simulink model "estimator_de_stare"  (R2023b)
settings: Solver=VariableStepAuto  StartTime=0.0  StopTime=1000  RelTol=1e-3
settings Model: Creator=Iustin  LastModifiedBy=Iustin

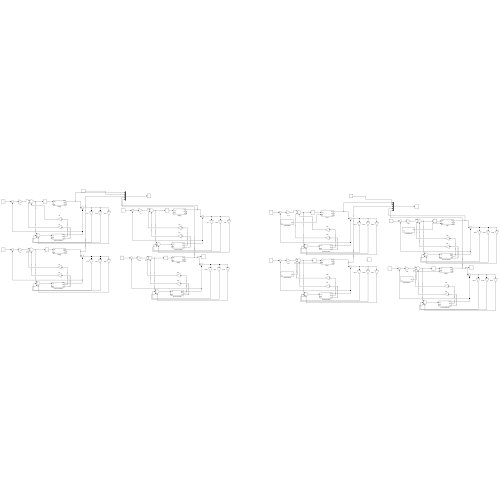
[thumbnail: Simulink's stored preview of the top-level diagram]
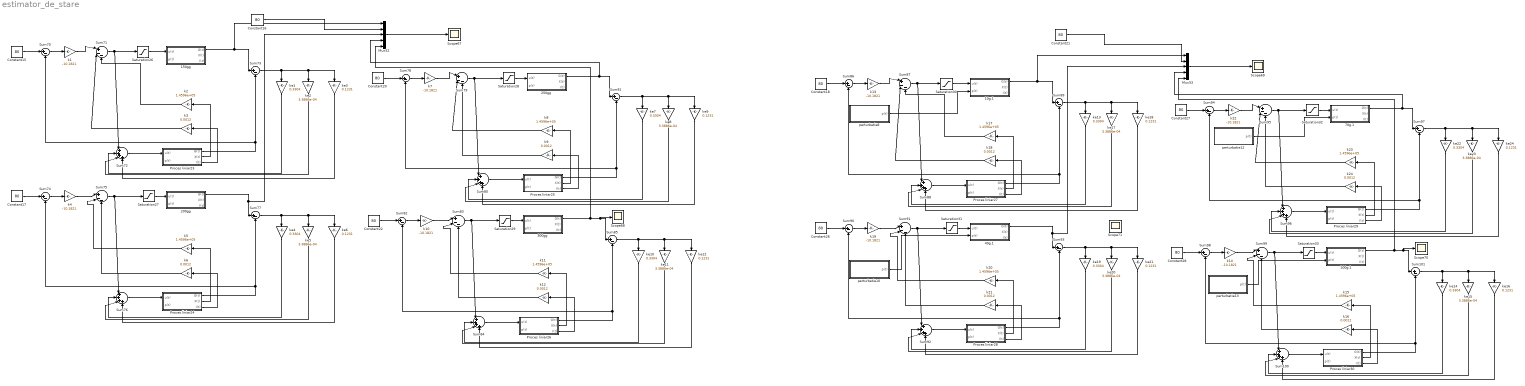
== system estimator_de_stare ==
  " Proces liniar23" : Subsystem  mask{p1=0.005, p2=0.017, p3=0.00000808, n=0.175, V=120, Gb=80, G0=100, Xb=0.0054}
  " Proces liniar24" : Subsystem  mask{p1=0.005, p2=0.017, p3=0.00000808, n=0.175, V=120, Gb=80, G0=100, Xb=0.0054}
  " Proces liniar25" : Subsystem  mask{p1=0.005, p2=0.017, p3=0.00000808, n=0.175, V=120, Gb=80, G0=100, Xb=0.0054}
  " Proces liniar26" : Subsystem  mask{p1=0.005, p2=0.017, p3=0.00000808, n=0.175, V=120, Gb=80, G0=100, Xb=0.0054}
  " Proces liniar27" : Subsystem  mask{p1=0.005, p2=0.017, p3=0.00000808, n=0.175, V=120, Gb=80, G0=100, Xb=0.0054}
  " Proces liniar28" : Subsystem  mask{p1=0.005, p2=0.017, p3=0.00000808, n=0.175, V=120, Gb=80, G0=100, Xb=0.0054}
  " Proces liniar29" : Subsystem  mask{p1=0.005, p2=0.017, p3=0.00000808, n=0.175, V=120, Gb=80, G0=100, Xb=0.0054}
  " Proces liniar30" : Subsystem  mask{p1=0.005, p2=0.017, p3=0.00000808, n=0.175, V=120, Gb=80, G0=100, Xb=0.0054}
  100g.1 : Subsystem  mask{p1=0.005, p2=0.017, p3=0.00000808, n=0.175, V=120, Gb=80, G0=100}
  10g.1 : Subsystem  mask{p1=0.005, p2=0.017, p3=0.00000808, n=0.175, V=120, Gb=80, G0=100}
  150gg : Subsystem  mask{p1=0.005, p2=0.017, p3=0.00000808, n=0.175, V=120, Gb=80, G0=150}
  200gg : Subsystem  mask{p1=0.005, p2=0.017, p3=0.00000808, n=0.175, V=120, Gb=80, G0=200}
  250gg : Subsystem  mask{p1=0.005, p2=0.017, p3=0.00000808, n=0.175, V=120, Gb=80, G0=250}
  300gg : Subsystem  mask{p1=0.005, p2=0.017, p3=0.00000808, n=0.175, V=120, Gb=80, G0=300}
  40g.1 : Subsystem  mask{p1=0.005, p2=0.017, p3=0.00000808, n=0.175, V=120, Gb=80, G0=100}
  70g.1 : Subsystem  mask{p1=0.005, p2=0.017, p3=0.00000808, n=0.175, V=120, Gb=80, G0=100}
  Constant{15..18,20..22,26..28} (10 alike) : Constant  Value=80
  Mux52 : Mux  Inputs=5
  Mux53 : Mux  Inputs=5
  Saturation{26..33} (8 alike) : Saturate  UpperLimit=500  LowerLimit=0
  Scope{67..71} (5 alike) : Scope
  Sum{72,76,80,84,88,92,96,100} (8 alike) : Sum  Inputs=|++++
  Sum{70,73..74,77..78,81..82,85..86,89..90,93..94,97..98,101} (16 alike) : Sum  Inputs=|+-
  Sum{71,75,79,83,87,91,95,99} (8 alike) : Sum  Inputs=|+--
  k{1,4,7,10,13..14,19,22} (8 alike) : Gain  Gain=-10.1821
  k{2,5,8,11,15,17,20,23} (8 alike) : Gain  Gain=1.4596e+05
  k{3,6,9,12,16,18,21,24} (8 alike) : Gain  Gain=0.0012
  ke{1,4,7,10,13..14,19,22} (8 alike) : Gain  Gain=0.3304
  ke{2,5,8,11,15,17,20,23} (8 alike) : Gain  Gain=3.3886e-04
  ke{3,6,9,12,16,18,21,24} (8 alike) : Gain  Gain=0.1231
  perturbatie10 : Subsystem  mask{Dg=40*1000, Ag=0.8, tg_max=40}
  perturbatie12 : Subsystem  mask{Dg=70*1000, Ag=0.8, tg_max=40}
  perturbatie13 : Subsystem  mask{Dg=100*1000, Ag=0.8, tg_max=40}
  perturbatie8 : Subsystem  mask{Dg=10*1000, Ag=0.8, tg_max=40}
  wires:
  ke17/1 -> Sum88/3
  ke19/1 -> Sum92/2
  k23/1 -> Sum95/2
  ke15/1 -> Sum100/3
  " Proces liniar28"/2(X(t)) -> k20/1
  " Proces liniar27"/1(" G(t)") -> Sum86/2, Sum89/2
  k17/1 -> Sum87/3
  " Proces liniar25"/2(X(t)) -> k8/1
  Constant18/1 -> Sum86/1
  " Proces liniar25"/3(I(t)) -> k9/1
  perturbatie10/1(p(t)) -> 40g.1/2(p(t))
  " Proces liniar26"/1(" G(t)") -> Sum82/2, Sum85/2
  k15/1 -> Sum99/2
  k22/1 -> Sum95/1
  ke2/1 -> Sum72/3
  k8/1 -> Sum79/2
  ke13/1 -> Sum88/2
  ke5/1 -> Sum76/3
  40g.1/1(" G(t)") -> Mux53/3, Sum93/1
  Sum75/1 -> Saturation27/1, Sum76/1
  Constant20/1 -> Sum78/1
  k11/1 -> Sum83/2
  Constant15/1 -> Sum70/1
  Constant28/1 -> Sum98/1
  " Proces liniar28"/3(I(t)) -> k21/1
  " Proces liniar29"/1(" G(t)") -> Sum94/2, Sum97/2
  ke7/1 -> Sum80/2
  10g.1/1(" G(t)") -> Mux53/1, Sum89/1
  Sum74/1 -> k4/1
  Sum86/1 -> k13/1
  Sum95/1 -> Saturation32/1, Sum96/1
  perturbatie13/1(p(t)) -> 100g.1/2(p(t))
  perturbatie12/1(p(t)) -> 70g.1/2(p(t))
  Sum93/1 -> ke19/1, ke20/1, ke21/1
  perturbatie8/1(p(t)) -> 10g.1/2(p(t))
  " Proces liniar27"/2(X(t)) -> k17/1
  Sum82/1 -> k10/1
  k19/1 -> Sum91/1
  ke14/1 -> Sum100/2
  " Proces liniar25"/1(" G(t)") -> Sum78/2, Sum81/2
  Constant26/1 -> Sum90/1
  Saturation31/1 -> 40g.1/1(" u(t)")
  ke22/1 -> Sum96/2
  ke20/1 -> Sum92/3
  ke10/1 -> Sum84/2
  k3/1 -> Sum71/2
  Constant27/1 -> Sum94/1
  Saturation32/1 -> 70g.1/1(" u(t)")
  ke23/1 -> Sum96/3
  Sum92/1 -> " Proces liniar28"/1(" u(t)")
  Sum88/1 -> " Proces liniar27"/1(" u(t)")
  " Proces liniar29"/3(I(t)) -> k24/1
  " Proces liniar27"/3(I(t)) -> k18/1
  Constant16/1 -> Mux52/2
  Saturation33/1 -> 100g.1/1(" u(t)")
  k21/1 -> Sum91/3
  k16/1 -> Sum99/3
  " Proces liniar29"/2(X(t)) -> k23/1
  Sum91/1 -> Saturation31/1, Sum92/1
  k9/1 -> Sum79/3
  Sum100/1 -> " Proces liniar30"/1(" u(t)")
  Sum89/1 -> ke13/1, ke17/1, ke18/1
  k6/1 -> Sum75/3
  ke24/1 -> Sum96/4
  ke21/1 -> Sum92/4
  ke16/1 -> Sum100/4
  Sum94/1 -> k22/1
  " Proces liniar30"/3(I(t)) -> k16/1
  Sum99/1 -> Saturation33/1, Sum100/1
  " Proces liniar30"/1(" G(t)") -> Sum98/2, Sum101/2
  k20/1 -> Sum91/2
  k24/1 -> Sum95/3
  Sum101/1 -> ke14/1, ke15/1, ke16/1
  Sum87/1 -> Saturation30/1, Sum88/1
  ke11/1 -> Sum84/3
  Mux53/1 -> Scope69/1
  k18/1 -> Sum87/2
  300gg/1(" G(t)") -> Mux52/5, Scope68/1, Sum85/1
  150gg/1(" G(t)") -> Mux52/1, Sum73/1
  k14/1 -> Sum99/1
  100g.1/1(" G(t)") -> Mux53/5, Scope70/1, Sum101/1
  k12/1 -> Sum83/3
  Sum77/1 -> ke4/1, ke5/1, ke6/1
  ke4/1 -> Sum76/2
  ke6/1 -> Sum76/4
  " Proces liniar24"/2(X(t)) -> k5/1
  Sum97/1 -> ke22/1, ke23/1, ke24/1
  Saturation27/1 -> 200gg/1(" u(t)")
  Constant17/1 -> Sum74/1
  ke12/1 -> Sum84/4
  " Proces liniar24"/3(I(t)) -> k6/1
  Sum98/1 -> k14/1
  Constant21/1 -> Mux53/2
  " Proces liniar26"/2(X(t)) -> k11/1
  " Proces liniar23"/1(" G(t)") -> Sum70/2, Sum73/2
  ke18/1 -> Sum88/4
  " Proces liniar28"/1(" G(t)") -> Sum90/2, Sum93/2
  " Proces liniar23"/2(X(t)) -> k2/1
  Sum76/1 -> " Proces liniar24"/1(" u(t)")
  Saturation30/1 -> 10g.1/1(" u(t)")
  200gg/1(" G(t)") -> Mux52/3, Sum77/1
  Sum90/1 -> k19/1
  " Proces liniar23"/3(I(t)) -> k3/1
  Sum71/1 -> Saturation26/1, Sum72/1
  Mux52/1 -> Scope67/1
  k5/1 -> Sum75/2
  k1/1 -> Sum71/1
  Sum70/1 -> k1/1
  Saturation28/1 -> 250gg/1(" u(t)")
  " Proces liniar26"/3(I(t)) -> k12/1
  Saturation29/1 -> 300gg/1(" u(t)")
  Sum84/1 -> " Proces liniar26"/1(" u(t)")
  70g.1/1(" G(t)") -> Mux53/4, Sum97/1
  Sum85/1 -> ke10/1, ke11/1, ke12/1
  " Proces liniar30"/2(X(t)) -> k15/1
  Sum73/1 -> ke1/1, ke2/1, ke3/1
  k2/1 -> Sum71/3
  Sum96/1 -> " Proces liniar29"/1(" u(t)")
  ke9/1 -> Sum80/4
  Constant22/1 -> Sum82/1
  k10/1 -> Sum83/1
  Sum78/1 -> k7/1
  ke3/1 -> Sum72/4
  Sum80/1 -> " Proces liniar25"/1(" u(t)")
  Saturation26/1 -> 150gg/1(" u(t)")
  ke8/1 -> Sum80/3
  Sum81/1 -> ke7/1, ke8/1, ke9/1
  Sum79/1 -> Saturation28/1, Sum80/1
  k13/1 -> Sum87/1
  Sum83/1 -> Saturation29/1, Sum84/1
  250gg/1(" G(t)") -> Mux52/4, Sum81/1
  ke1/1 -> Sum72/2
  " Proces liniar24"/1(" G(t)") -> Sum74/2, Sum77/2
  k4/1 -> Sum75/1
  k7/1 -> Sum79/1
  Sum72/1 -> " Proces liniar23"/1(" u(t)")

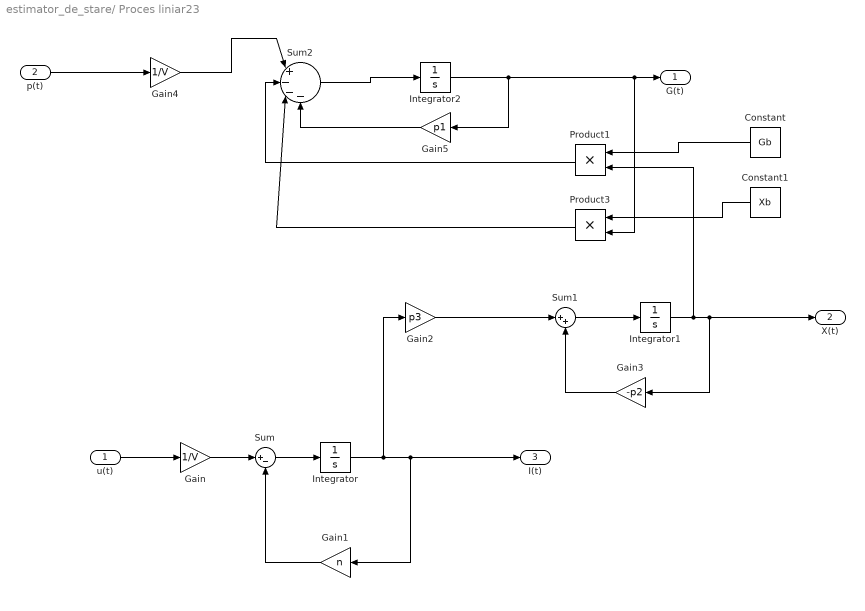
== system estimator_de_stare/ Proces liniar23 ==
  " u(t)" : Inport
  p(t) : Inport  Port=2
  Constant : Constant  Value=Gb
  Constant1 : Constant  Value=Xb
  Gain : Gain  Gain=1/V
  Gain1 : Gain  Gain=n
  Gain2 : Gain  Gain=p3
  Gain3 : Gain  Gain=-p2
  Gain4 : Gain  Gain=1/V
  Gain5 : Gain  Gain=p1
  Integrator : Integrator
  Integrator1 : Integrator
  Integrator2 : Integrator  InitialCondition=G0
  Product1 : Product
  Product3 : Product
  Sum : Sum  Inputs=|+-
  Sum1 : Sum  Inputs=|++
  Sum2 : Sum  Inputs=|+---
  " G(t)" : Outport
  X(t) : Outport  Port=2
  I(t) : Outport  Port=3
  wires:
  Gain2/1 -> Sum1/1
  Gain/1 -> Sum/1
  " u(t)"/1 -> Gain/1
  Sum/1 -> Integrator/1
  Gain1/1 -> Sum/2
  Integrator2/1 -> Product3/2, " G(t)"/1, Gain5/1
  Integrator1/1 -> Product1/2, Gain3/1, X(t)/1
  Integrator/1 -> Gain2/1, I(t)/1, Gain1/1
  Gain3/1 -> Sum1/2
  Gain4/1 -> Sum2/1
  Gain5/1 -> Sum2/4
  p(t)/1 -> Gain4/1
  Sum1/1 -> Integrator1/1
  Sum2/1 -> Integrator2/1
  Constant/1 -> Product1/1
  Constant1/1 -> Product3/1
  Product3/1 -> Sum2/3
  Product1/1 -> Sum2/2

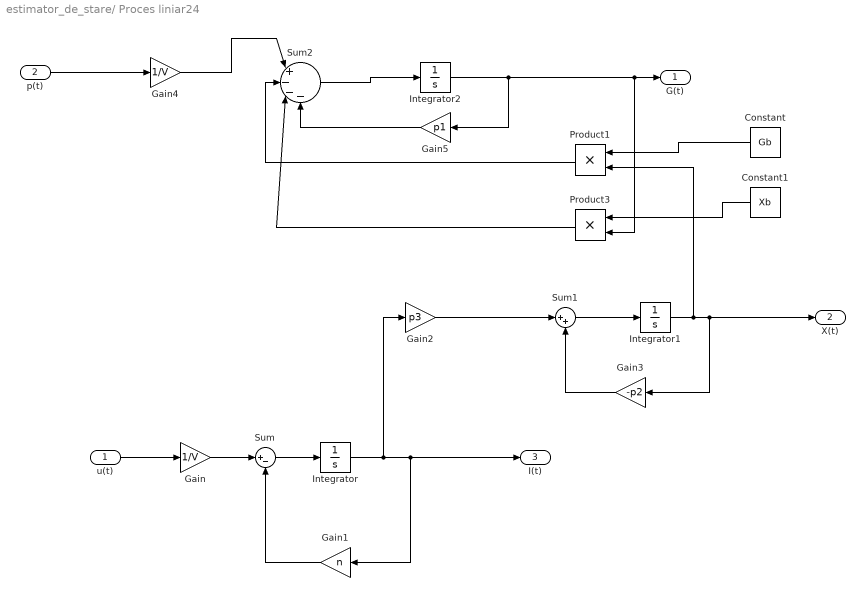
== system estimator_de_stare/ Proces liniar24 ==
  " u(t)" : Inport
  p(t) : Inport  Port=2
  Constant : Constant  Value=Gb
  Constant1 : Constant  Value=Xb
  Gain : Gain  Gain=1/V
  Gain1 : Gain  Gain=n
  Gain2 : Gain  Gain=p3
  Gain3 : Gain  Gain=-p2
  Gain4 : Gain  Gain=1/V
  Gain5 : Gain  Gain=p1
  Integrator : Integrator
  Integrator1 : Integrator
  Integrator2 : Integrator  InitialCondition=G0
  Product1 : Product
  Product3 : Product
  Sum : Sum  Inputs=|+-
  Sum1 : Sum  Inputs=|++
  Sum2 : Sum  Inputs=|+---
  " G(t)" : Outport
  X(t) : Outport  Port=2
  I(t) : Outport  Port=3
  wires:
  Gain2/1 -> Sum1/1
  Gain/1 -> Sum/1
  " u(t)"/1 -> Gain/1
  Sum/1 -> Integrator/1
  Gain1/1 -> Sum/2
  Integrator2/1 -> Product3/2, " G(t)"/1, Gain5/1
  Integrator1/1 -> Product1/2, Gain3/1, X(t)/1
  Integrator/1 -> Gain2/1, I(t)/1, Gain1/1
  Gain3/1 -> Sum1/2
  Gain4/1 -> Sum2/1
  Gain5/1 -> Sum2/4
  p(t)/1 -> Gain4/1
  Sum1/1 -> Integrator1/1
  Sum2/1 -> Integrator2/1
  Constant/1 -> Product1/1
  Constant1/1 -> Product3/1
  Product3/1 -> Sum2/3
  Product1/1 -> Sum2/2

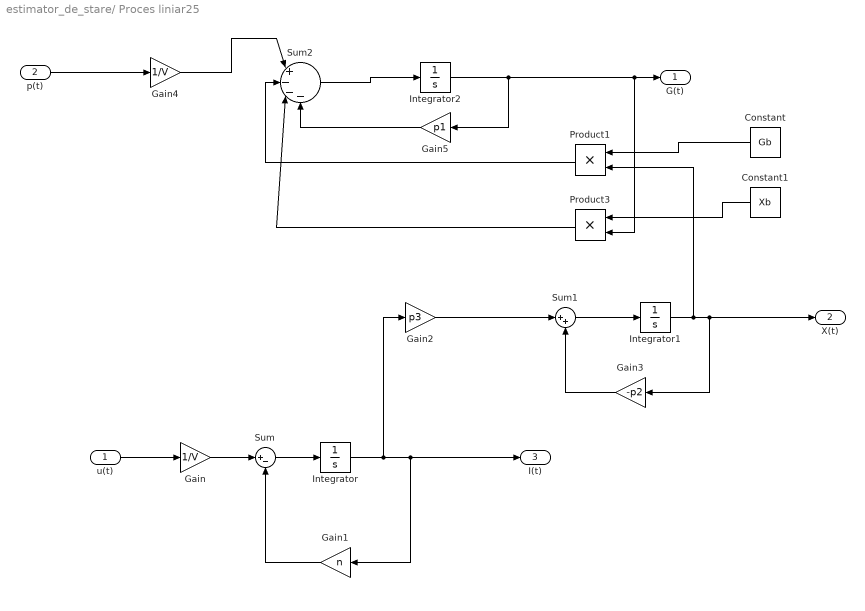
== system estimator_de_stare/ Proces liniar25 ==
  " u(t)" : Inport
  p(t) : Inport  Port=2
  Constant : Constant  Value=Gb
  Constant1 : Constant  Value=Xb
  Gain : Gain  Gain=1/V
  Gain1 : Gain  Gain=n
  Gain2 : Gain  Gain=p3
  Gain3 : Gain  Gain=-p2
  Gain4 : Gain  Gain=1/V
  Gain5 : Gain  Gain=p1
  Integrator : Integrator
  Integrator1 : Integrator
  Integrator2 : Integrator  InitialCondition=G0
  Product1 : Product
  Product3 : Product
  Sum : Sum  Inputs=|+-
  Sum1 : Sum  Inputs=|++
  Sum2 : Sum  Inputs=|+---
  " G(t)" : Outport
  X(t) : Outport  Port=2
  I(t) : Outport  Port=3
  wires:
  Gain2/1 -> Sum1/1
  Gain/1 -> Sum/1
  " u(t)"/1 -> Gain/1
  Sum/1 -> Integrator/1
  Gain1/1 -> Sum/2
  Integrator2/1 -> Product3/2, " G(t)"/1, Gain5/1
  Integrator1/1 -> Product1/2, Gain3/1, X(t)/1
  Integrator/1 -> Gain2/1, I(t)/1, Gain1/1
  Gain3/1 -> Sum1/2
  Gain4/1 -> Sum2/1
  Gain5/1 -> Sum2/4
  p(t)/1 -> Gain4/1
  Sum1/1 -> Integrator1/1
  Sum2/1 -> Integrator2/1
  Constant/1 -> Product1/1
  Constant1/1 -> Product3/1
  Product3/1 -> Sum2/3
  Product1/1 -> Sum2/2

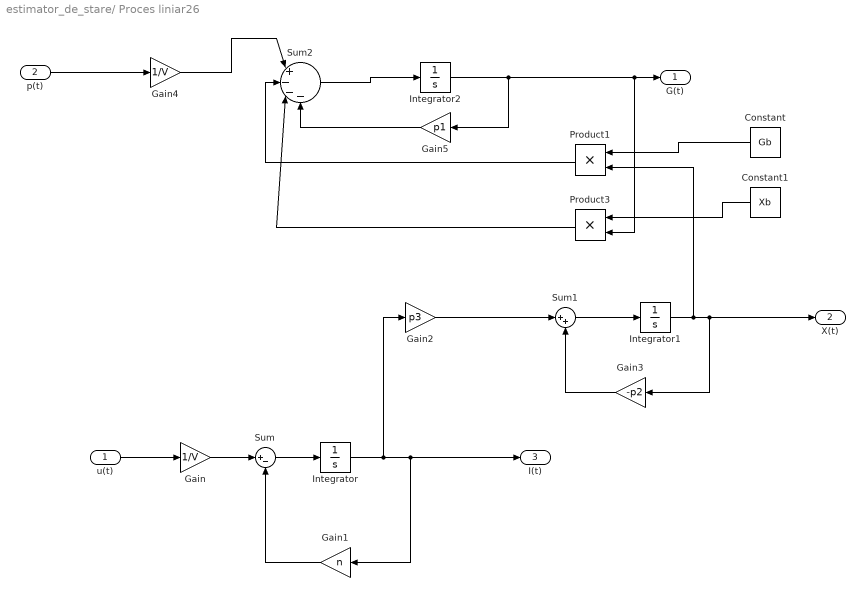
== system estimator_de_stare/ Proces liniar26 ==
  " u(t)" : Inport
  p(t) : Inport  Port=2
  Constant : Constant  Value=Gb
  Constant1 : Constant  Value=Xb
  Gain : Gain  Gain=1/V
  Gain1 : Gain  Gain=n
  Gain2 : Gain  Gain=p3
  Gain3 : Gain  Gain=-p2
  Gain4 : Gain  Gain=1/V
  Gain5 : Gain  Gain=p1
  Integrator : Integrator
  Integrator1 : Integrator
  Integrator2 : Integrator  InitialCondition=G0
  Product1 : Product
  Product3 : Product
  Sum : Sum  Inputs=|+-
  Sum1 : Sum  Inputs=|++
  Sum2 : Sum  Inputs=|+---
  " G(t)" : Outport
  X(t) : Outport  Port=2
  I(t) : Outport  Port=3
  wires:
  Gain2/1 -> Sum1/1
  Gain/1 -> Sum/1
  " u(t)"/1 -> Gain/1
  Sum/1 -> Integrator/1
  Gain1/1 -> Sum/2
  Integrator2/1 -> Product3/2, " G(t)"/1, Gain5/1
  Integrator1/1 -> Product1/2, Gain3/1, X(t)/1
  Integrator/1 -> Gain2/1, I(t)/1, Gain1/1
  Gain3/1 -> Sum1/2
  Gain4/1 -> Sum2/1
  Gain5/1 -> Sum2/4
  p(t)/1 -> Gain4/1
  Sum1/1 -> Integrator1/1
  Sum2/1 -> Integrator2/1
  Constant/1 -> Product1/1
  Constant1/1 -> Product3/1
  Product3/1 -> Sum2/3
  Product1/1 -> Sum2/2

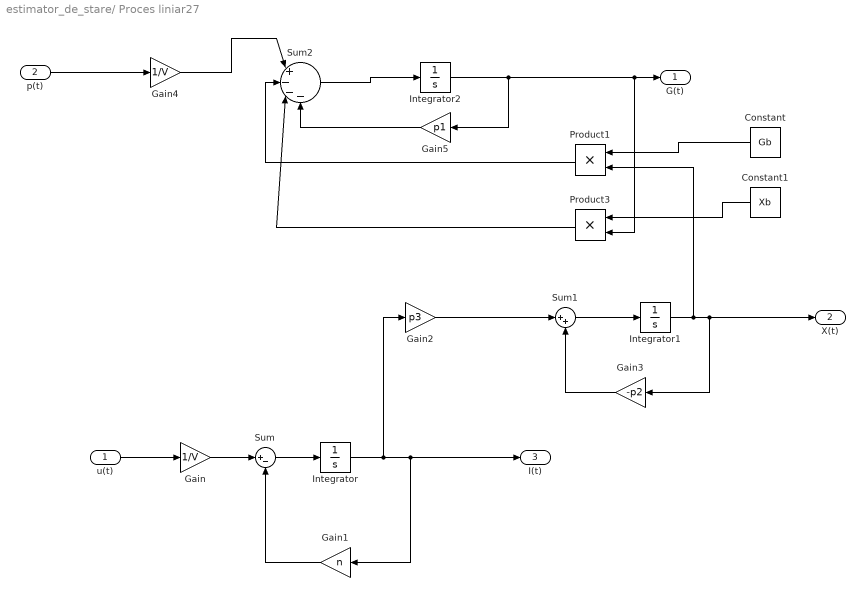
== system estimator_de_stare/ Proces liniar27 ==
  " u(t)" : Inport
  p(t) : Inport  Port=2
  Constant : Constant  Value=Gb
  Constant1 : Constant  Value=Xb
  Gain : Gain  Gain=1/V
  Gain1 : Gain  Gain=n
  Gain2 : Gain  Gain=p3
  Gain3 : Gain  Gain=-p2
  Gain4 : Gain  Gain=1/V
  Gain5 : Gain  Gain=p1
  Integrator : Integrator
  Integrator1 : Integrator
  Integrator2 : Integrator  InitialCondition=G0
  Product1 : Product
  Product3 : Product
  Sum : Sum  Inputs=|+-
  Sum1 : Sum  Inputs=|++
  Sum2 : Sum  Inputs=|+---
  " G(t)" : Outport
  X(t) : Outport  Port=2
  I(t) : Outport  Port=3
  wires:
  Gain2/1 -> Sum1/1
  Gain/1 -> Sum/1
  " u(t)"/1 -> Gain/1
  Sum/1 -> Integrator/1
  Gain1/1 -> Sum/2
  Integrator2/1 -> Product3/2, " G(t)"/1, Gain5/1
  Integrator1/1 -> Product1/2, Gain3/1, X(t)/1
  Integrator/1 -> Gain2/1, I(t)/1, Gain1/1
  Gain3/1 -> Sum1/2
  Gain4/1 -> Sum2/1
  Gain5/1 -> Sum2/4
  p(t)/1 -> Gain4/1
  Sum1/1 -> Integrator1/1
  Sum2/1 -> Integrator2/1
  Constant/1 -> Product1/1
  Constant1/1 -> Product3/1
  Product3/1 -> Sum2/3
  Product1/1 -> Sum2/2

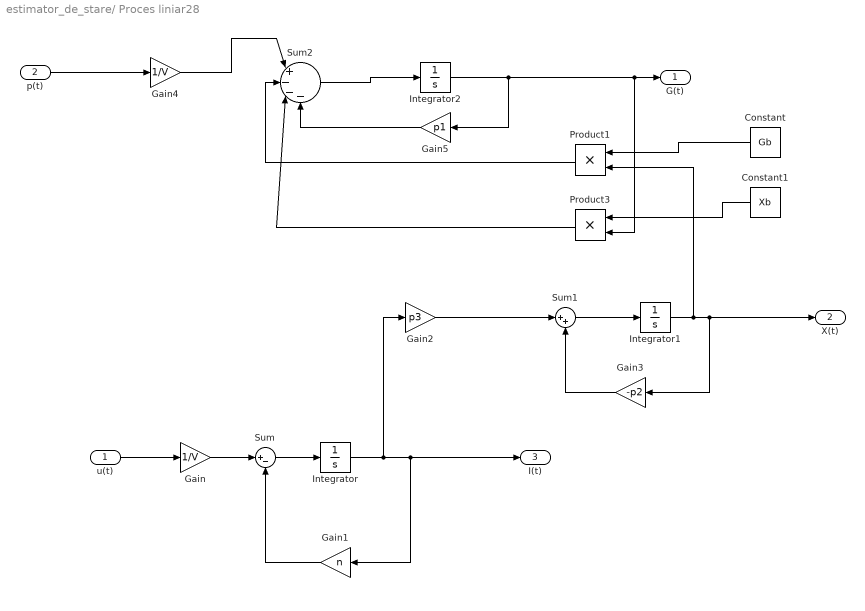
== system estimator_de_stare/ Proces liniar28 ==
  " u(t)" : Inport
  p(t) : Inport  Port=2
  Constant : Constant  Value=Gb
  Constant1 : Constant  Value=Xb
  Gain : Gain  Gain=1/V
  Gain1 : Gain  Gain=n
  Gain2 : Gain  Gain=p3
  Gain3 : Gain  Gain=-p2
  Gain4 : Gain  Gain=1/V
  Gain5 : Gain  Gain=p1
  Integrator : Integrator
  Integrator1 : Integrator
  Integrator2 : Integrator  InitialCondition=G0
  Product1 : Product
  Product3 : Product
  Sum : Sum  Inputs=|+-
  Sum1 : Sum  Inputs=|++
  Sum2 : Sum  Inputs=|+---
  " G(t)" : Outport
  X(t) : Outport  Port=2
  I(t) : Outport  Port=3
  wires:
  Gain2/1 -> Sum1/1
  Gain/1 -> Sum/1
  " u(t)"/1 -> Gain/1
  Sum/1 -> Integrator/1
  Gain1/1 -> Sum/2
  Integrator2/1 -> Product3/2, " G(t)"/1, Gain5/1
  Integrator1/1 -> Product1/2, Gain3/1, X(t)/1
  Integrator/1 -> Gain2/1, I(t)/1, Gain1/1
  Gain3/1 -> Sum1/2
  Gain4/1 -> Sum2/1
  Gain5/1 -> Sum2/4
  p(t)/1 -> Gain4/1
  Sum1/1 -> Integrator1/1
  Sum2/1 -> Integrator2/1
  Constant/1 -> Product1/1
  Constant1/1 -> Product3/1
  Product3/1 -> Sum2/3
  Product1/1 -> Sum2/2

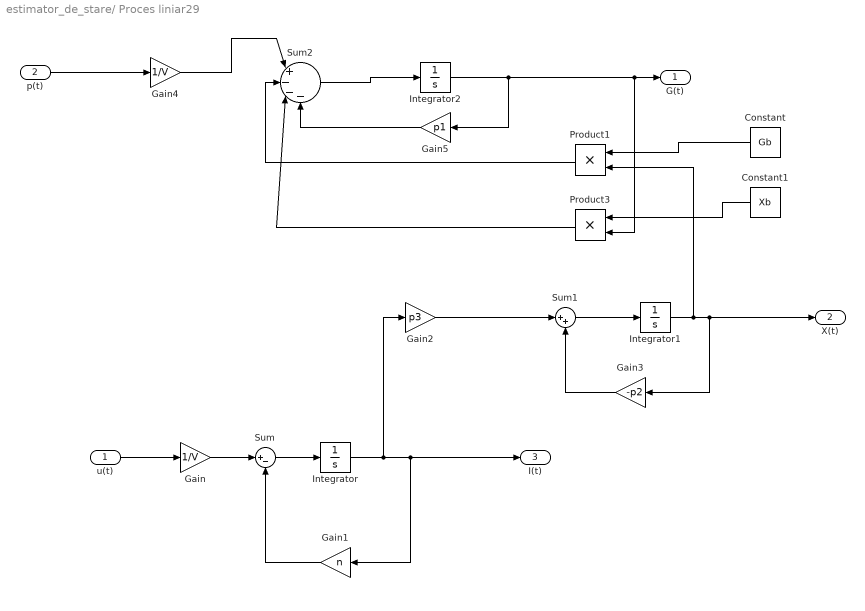
== system estimator_de_stare/ Proces liniar29 ==
  " u(t)" : Inport
  p(t) : Inport  Port=2
  Constant : Constant  Value=Gb
  Constant1 : Constant  Value=Xb
  Gain : Gain  Gain=1/V
  Gain1 : Gain  Gain=n
  Gain2 : Gain  Gain=p3
  Gain3 : Gain  Gain=-p2
  Gain4 : Gain  Gain=1/V
  Gain5 : Gain  Gain=p1
  Integrator : Integrator
  Integrator1 : Integrator
  Integrator2 : Integrator  InitialCondition=G0
  Product1 : Product
  Product3 : Product
  Sum : Sum  Inputs=|+-
  Sum1 : Sum  Inputs=|++
  Sum2 : Sum  Inputs=|+---
  " G(t)" : Outport
  X(t) : Outport  Port=2
  I(t) : Outport  Port=3
  wires:
  Gain2/1 -> Sum1/1
  Gain/1 -> Sum/1
  " u(t)"/1 -> Gain/1
  Sum/1 -> Integrator/1
  Gain1/1 -> Sum/2
  Integrator2/1 -> Product3/2, " G(t)"/1, Gain5/1
  Integrator1/1 -> Product1/2, Gain3/1, X(t)/1
  Integrator/1 -> Gain2/1, I(t)/1, Gain1/1
  Gain3/1 -> Sum1/2
  Gain4/1 -> Sum2/1
  Gain5/1 -> Sum2/4
  p(t)/1 -> Gain4/1
  Sum1/1 -> Integrator1/1
  Sum2/1 -> Integrator2/1
  Constant/1 -> Product1/1
  Constant1/1 -> Product3/1
  Product3/1 -> Sum2/3
  Product1/1 -> Sum2/2

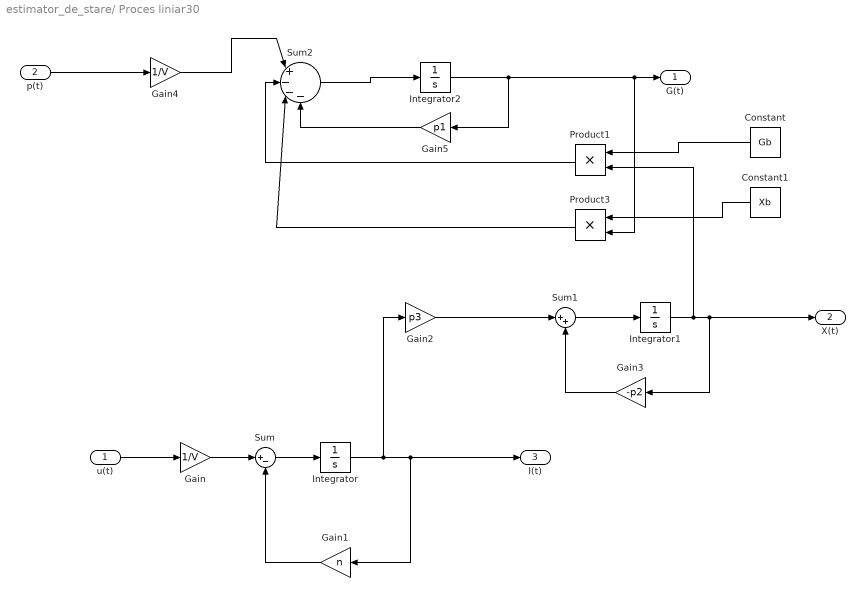
== system estimator_de_stare/ Proces liniar30 ==
  " u(t)" : Inport
  p(t) : Inport  Port=2
  Constant : Constant  Value=Gb
  Constant1 : Constant  Value=Xb
  Gain : Gain  Gain=1/V
  Gain1 : Gain  Gain=n
  Gain2 : Gain  Gain=p3
  Gain3 : Gain  Gain=-p2
  Gain4 : Gain  Gain=1/V
  Gain5 : Gain  Gain=p1
  Integrator : Integrator
  Integrator1 : Integrator
  Integrator2 : Integrator  InitialCondition=G0
  Product1 : Product
  Product3 : Product
  Sum : Sum  Inputs=|+-
  Sum1 : Sum  Inputs=|++
  Sum2 : Sum  Inputs=|+---
  " G(t)" : Outport
  X(t) : Outport  Port=2
  I(t) : Outport  Port=3
  wires:
  Gain2/1 -> Sum1/1
  Gain/1 -> Sum/1
  " u(t)"/1 -> Gain/1
  Sum/1 -> Integrator/1
  Gain1/1 -> Sum/2
  Integrator2/1 -> Product3/2, " G(t)"/1, Gain5/1
  Integrator1/1 -> Product1/2, Gain3/1, X(t)/1
  Integrator/1 -> Gain2/1, I(t)/1, Gain1/1
  Gain3/1 -> Sum1/2
  Gain4/1 -> Sum2/1
  Gain5/1 -> Sum2/4
  p(t)/1 -> Gain4/1
  Sum1/1 -> Integrator1/1
  Sum2/1 -> Integrator2/1
  Constant/1 -> Product1/1
  Constant1/1 -> Product3/1
  Product3/1 -> Sum2/3
  Product1/1 -> Sum2/2

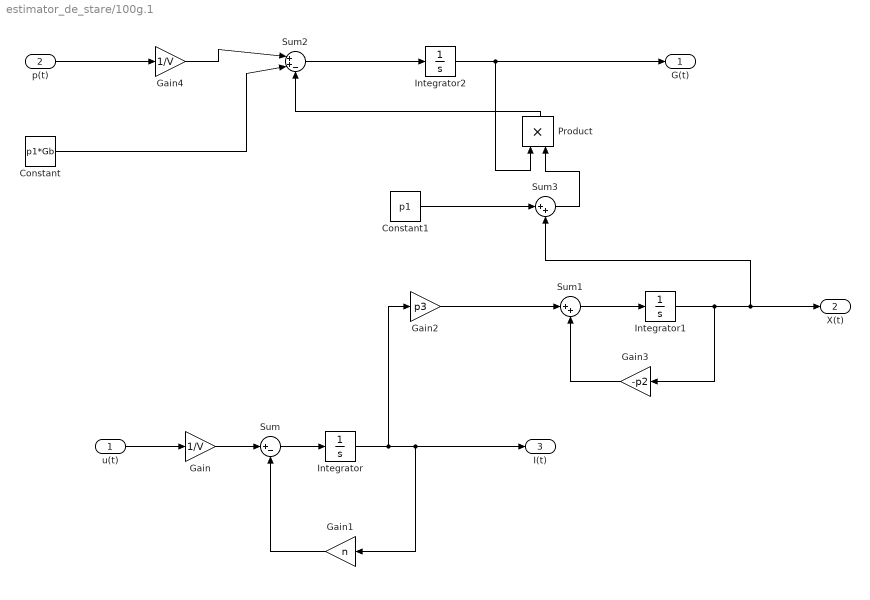
== system estimator_de_stare/100g.1 ==
  " u(t)" : Inport
  p(t) : Inport  Port=2
  Constant : Constant  Value=p1*Gb
  Constant1 : Constant  Value=p1
  Gain : Gain  Gain=1/V
  Gain1 : Gain  Gain=n
  Gain2 : Gain  Gain=p3
  Gain3 : Gain  Gain=-p2
  Gain4 : Gain  Gain=1/V
  Integrator : Integrator
  Integrator1 : Integrator
  Integrator2 : Integrator  InitialCondition=G0
  Product : Product
  Sum : Sum  Inputs=|+-
  Sum1 : Sum  Inputs=|++
  Sum2 : Sum  Inputs=|++-
  Sum3 : Sum  Inputs=|++
  " G(t)" : Outport
  X(t) : Outport  Port=2
  I(t) : Outport  Port=3
  wires:
  " u(t)"/1 -> Gain/1
  Gain/1 -> Sum/1
  Sum/1 -> Integrator/1
  Integrator/1 -> Gain2/1, I(t)/1, Gain1/1
  Gain1/1 -> Sum/2
  Gain2/1 -> Sum1/1
  Gain3/1 -> Sum1/2
  Integrator1/1 -> Gain3/1, Sum3/2, X(t)/1
  p(t)/1 -> Gain4/1
  Gain4/1 -> Sum2/1
  Constant/1 -> Sum2/2
  Constant1/1 -> Sum3/1
  Sum2/1 -> Integrator2/1
  Product/1 -> Sum2/3
  Sum3/1 -> Product/2
  Integrator2/1 -> Product/1, " G(t)"/1
  Sum1/1 -> Integrator1/1

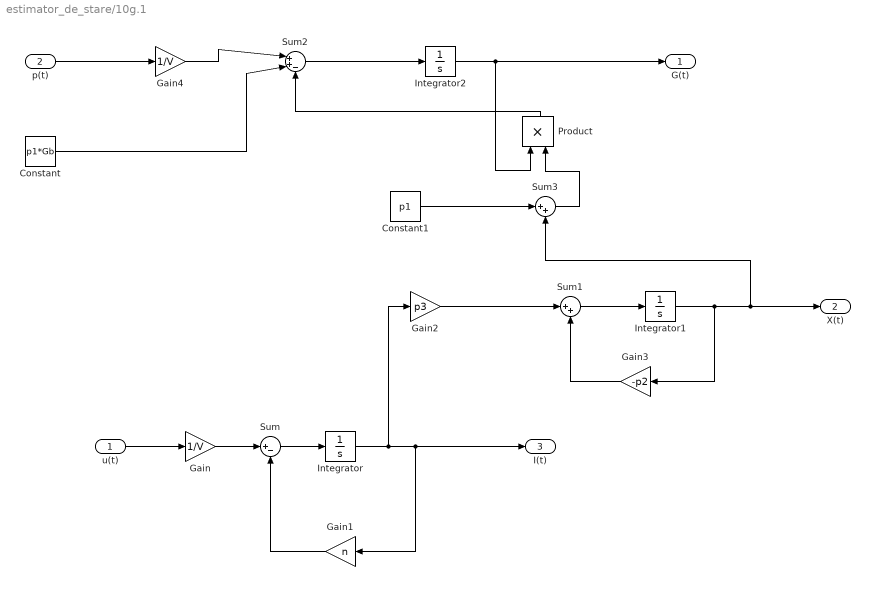
== system estimator_de_stare/10g.1 ==
  " u(t)" : Inport
  p(t) : Inport  Port=2
  Constant : Constant  Value=p1*Gb
  Constant1 : Constant  Value=p1
  Gain : Gain  Gain=1/V
  Gain1 : Gain  Gain=n
  Gain2 : Gain  Gain=p3
  Gain3 : Gain  Gain=-p2
  Gain4 : Gain  Gain=1/V
  Integrator : Integrator
  Integrator1 : Integrator
  Integrator2 : Integrator  InitialCondition=G0
  Product : Product
  Sum : Sum  Inputs=|+-
  Sum1 : Sum  Inputs=|++
  Sum2 : Sum  Inputs=|++-
  Sum3 : Sum  Inputs=|++
  " G(t)" : Outport
  X(t) : Outport  Port=2
  I(t) : Outport  Port=3
  wires:
  " u(t)"/1 -> Gain/1
  Gain/1 -> Sum/1
  Sum/1 -> Integrator/1
  Integrator/1 -> Gain2/1, I(t)/1, Gain1/1
  Gain1/1 -> Sum/2
  Gain2/1 -> Sum1/1
  Gain3/1 -> Sum1/2
  Integrator1/1 -> Gain3/1, Sum3/2, X(t)/1
  p(t)/1 -> Gain4/1
  Gain4/1 -> Sum2/1
  Constant/1 -> Sum2/2
  Constant1/1 -> Sum3/1
  Sum2/1 -> Integrator2/1
  Product/1 -> Sum2/3
  Sum3/1 -> Product/2
  Integrator2/1 -> Product/1, " G(t)"/1
  Sum1/1 -> Integrator1/1

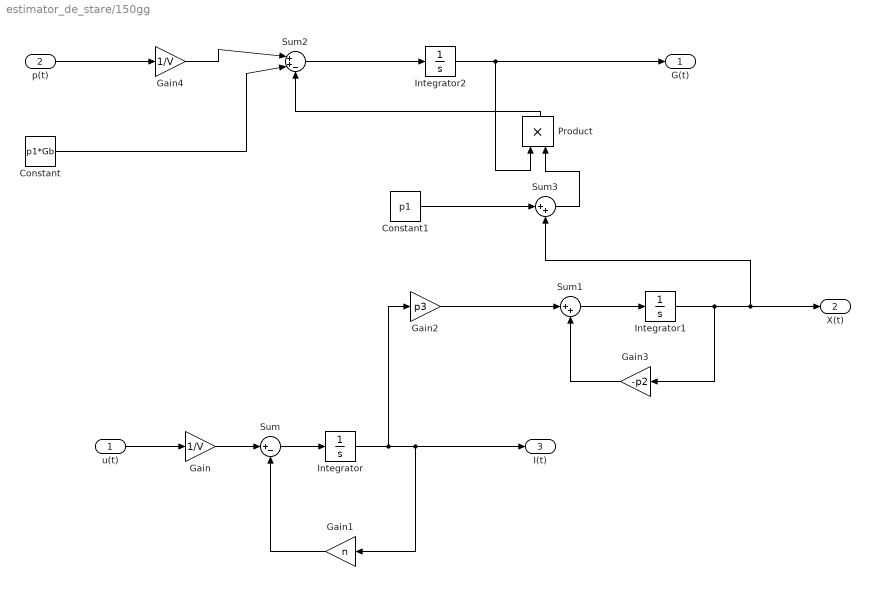
== system estimator_de_stare/150gg ==
  " u(t)" : Inport
  p(t) : Inport  Port=2
  Constant : Constant  Value=p1*Gb
  Constant1 : Constant  Value=p1
  Gain : Gain  Gain=1/V
  Gain1 : Gain  Gain=n
  Gain2 : Gain  Gain=p3
  Gain3 : Gain  Gain=-p2
  Gain4 : Gain  Gain=1/V
  Integrator : Integrator
  Integrator1 : Integrator
  Integrator2 : Integrator  InitialCondition=G0
  Product : Product
  Sum : Sum  Inputs=|+-
  Sum1 : Sum  Inputs=|++
  Sum2 : Sum  Inputs=|++-
  Sum3 : Sum  Inputs=|++
  " G(t)" : Outport
  X(t) : Outport  Port=2
  I(t) : Outport  Port=3
  wires:
  " u(t)"/1 -> Gain/1
  Gain/1 -> Sum/1
  Sum/1 -> Integrator/1
  Integrator/1 -> Gain2/1, I(t)/1, Gain1/1
  Gain1/1 -> Sum/2
  Gain2/1 -> Sum1/1
  Gain3/1 -> Sum1/2
  Integrator1/1 -> Gain3/1, Sum3/2, X(t)/1
  p(t)/1 -> Gain4/1
  Gain4/1 -> Sum2/1
  Constant/1 -> Sum2/2
  Constant1/1 -> Sum3/1
  Sum2/1 -> Integrator2/1
  Product/1 -> Sum2/3
  Sum3/1 -> Product/2
  Integrator2/1 -> Product/1, " G(t)"/1
  Sum1/1 -> Integrator1/1

== system estimator_de_stare/200gg ==
  " u(t)" : Inport
  p(t) : Inport  Port=2
  Constant : Constant  Value=p1*Gb
  Constant1 : Constant  Value=p1
  Gain : Gain  Gain=1/V
  Gain1 : Gain  Gain=n
  Gain2 : Gain  Gain=p3
  Gain3 : Gain  Gain=-p2
  Gain4 : Gain  Gain=1/V
  Integrator : Integrator
  Integrator1 : Integrator
  Integrator2 : Integrator  InitialCondition=G0
  Product : Product
  Sum : Sum  Inputs=|+-
  Sum1 : Sum  Inputs=|++
  Sum2 : Sum  Inputs=|++-
  Sum3 : Sum  Inputs=|++
  " G(t)" : Outport
  X(t) : Outport  Port=2
  I(t) : Outport  Port=3
  wires:
  " u(t)"/1 -> Gain/1
  Gain/1 -> Sum/1
  Sum/1 -> Integrator/1
  Integrator/1 -> Gain2/1, I(t)/1, Gain1/1
  Gain1/1 -> Sum/2
  Gain2/1 -> Sum1/1
  Gain3/1 -> Sum1/2
  Integrator1/1 -> Gain3/1, Sum3/2, X(t)/1
  p(t)/1 -> Gain4/1
  Gain4/1 -> Sum2/1
  Constant/1 -> Sum2/2
  Constant1/1 -> Sum3/1
  Sum2/1 -> Integrator2/1
  Product/1 -> Sum2/3
  Sum3/1 -> Product/2
  Integrator2/1 -> Product/1, " G(t)"/1
  Sum1/1 -> Integrator1/1

== system estimator_de_stare/250gg ==
  " u(t)" : Inport
  p(t) : Inport  Port=2
  Constant : Constant  Value=p1*Gb
  Constant1 : Constant  Value=p1
  Gain : Gain  Gain=1/V
  Gain1 : Gain  Gain=n
  Gain2 : Gain  Gain=p3
  Gain3 : Gain  Gain=-p2
  Gain4 : Gain  Gain=1/V
  Integrator : Integrator
  Integrator1 : Integrator
  Integrator2 : Integrator  InitialCondition=G0
  Product : Product
  Sum : Sum  Inputs=|+-
  Sum1 : Sum  Inputs=|++
  Sum2 : Sum  Inputs=|++-
  Sum3 : Sum  Inputs=|++
  " G(t)" : Outport
  X(t) : Outport  Port=2
  I(t) : Outport  Port=3
  wires:
  " u(t)"/1 -> Gain/1
  Gain/1 -> Sum/1
  Sum/1 -> Integrator/1
  Integrator/1 -> Gain2/1, I(t)/1, Gain1/1
  Gain1/1 -> Sum/2
  Gain2/1 -> Sum1/1
  Gain3/1 -> Sum1/2
  Integrator1/1 -> Gain3/1, Sum3/2, X(t)/1
  p(t)/1 -> Gain4/1
  Gain4/1 -> Sum2/1
  Constant/1 -> Sum2/2
  Constant1/1 -> Sum3/1
  Sum2/1 -> Integrator2/1
  Product/1 -> Sum2/3
  Sum3/1 -> Product/2
  Integrator2/1 -> Product/1, " G(t)"/1
  Sum1/1 -> Integrator1/1

== system estimator_de_stare/300gg ==
  " u(t)" : Inport
  p(t) : Inport  Port=2
  Constant : Constant  Value=p1*Gb
  Constant1 : Constant  Value=p1
  Gain : Gain  Gain=1/V
  Gain1 : Gain  Gain=n
  Gain2 : Gain  Gain=p3
  Gain3 : Gain  Gain=-p2
  Gain4 : Gain  Gain=1/V
  Integrator : Integrator
  Integrator1 : Integrator
  Integrator2 : Integrator  InitialCondition=G0
  Product : Product
  Sum : Sum  Inputs=|+-
  Sum1 : Sum  Inputs=|++
  Sum2 : Sum  Inputs=|++-
  Sum3 : Sum  Inputs=|++
  " G(t)" : Outport
  X(t) : Outport  Port=2
  I(t) : Outport  Port=3
  wires:
  " u(t)"/1 -> Gain/1
  Gain/1 -> Sum/1
  Sum/1 -> Integrator/1
  Integrator/1 -> Gain2/1, I(t)/1, Gain1/1
  Gain1/1 -> Sum/2
  Gain2/1 -> Sum1/1
  Gain3/1 -> Sum1/2
  Integrator1/1 -> Gain3/1, Sum3/2, X(t)/1
  p(t)/1 -> Gain4/1
  Gain4/1 -> Sum2/1
  Constant/1 -> Sum2/2
  Constant1/1 -> Sum3/1
  Sum2/1 -> Integrator2/1
  Product/1 -> Sum2/3
  Sum3/1 -> Product/2
  Integrator2/1 -> Product/1, " G(t)"/1
  Sum1/1 -> Integrator1/1

== system estimator_de_stare/40g.1 ==
  " u(t)" : Inport
  p(t) : Inport  Port=2
  Constant : Constant  Value=p1*Gb
  Constant1 : Constant  Value=p1
  Gain : Gain  Gain=1/V
  Gain1 : Gain  Gain=n
  Gain2 : Gain  Gain=p3
  Gain3 : Gain  Gain=-p2
  Gain4 : Gain  Gain=1/V
  Integrator : Integrator
  Integrator1 : Integrator
  Integrator2 : Integrator  InitialCondition=G0
  Product : Product
  Sum : Sum  Inputs=|+-
  Sum1 : Sum  Inputs=|++
  Sum2 : Sum  Inputs=|++-
  Sum3 : Sum  Inputs=|++
  " G(t)" : Outport
  X(t) : Outport  Port=2
  I(t) : Outport  Port=3
  wires:
  " u(t)"/1 -> Gain/1
  Gain/1 -> Sum/1
  Sum/1 -> Integrator/1
  Integrator/1 -> Gain2/1, I(t)/1, Gain1/1
  Gain1/1 -> Sum/2
  Gain2/1 -> Sum1/1
  Gain3/1 -> Sum1/2
  Integrator1/1 -> Gain3/1, Sum3/2, X(t)/1
  p(t)/1 -> Gain4/1
  Gain4/1 -> Sum2/1
  Constant/1 -> Sum2/2
  Constant1/1 -> Sum3/1
  Sum2/1 -> Integrator2/1
  Product/1 -> Sum2/3
  Sum3/1 -> Product/2
  Integrator2/1 -> Product/1, " G(t)"/1
  Sum1/1 -> Integrator1/1

== system estimator_de_stare/70g.1 ==
  " u(t)" : Inport
  p(t) : Inport  Port=2
  Constant : Constant  Value=p1*Gb
  Constant1 : Constant  Value=p1
  Gain : Gain  Gain=1/V
  Gain1 : Gain  Gain=n
  Gain2 : Gain  Gain=p3
  Gain3 : Gain  Gain=-p2
  Gain4 : Gain  Gain=1/V
  Integrator : Integrator
  Integrator1 : Integrator
  Integrator2 : Integrator  InitialCondition=G0
  Product : Product
  Sum : Sum  Inputs=|+-
  Sum1 : Sum  Inputs=|++
  Sum2 : Sum  Inputs=|++-
  Sum3 : Sum  Inputs=|++
  " G(t)" : Outport
  X(t) : Outport  Port=2
  I(t) : Outport  Port=3
  wires:
  " u(t)"/1 -> Gain/1
  Gain/1 -> Sum/1
  Sum/1 -> Integrator/1
  Integrator/1 -> Gain2/1, I(t)/1, Gain1/1
  Gain1/1 -> Sum/2
  Gain2/1 -> Sum1/1
  Gain3/1 -> Sum1/2
  Integrator1/1 -> Gain3/1, Sum3/2, X(t)/1
  p(t)/1 -> Gain4/1
  Gain4/1 -> Sum2/1
  Constant/1 -> Sum2/2
  Constant1/1 -> Sum3/1
  Sum2/1 -> Integrator2/1
  Product/1 -> Sum2/3
  Sum3/1 -> Product/2
  Integrator2/1 -> Product/1, " G(t)"/1
  Sum1/1 -> Integrator1/1

== system estimator_de_stare/perturbatie10 ==
  Clock : Clock
  Constant : Constant  Value=Dg
  Constant1 : Constant  Value=Ag
  Gain : Gain  Gain=-1/tg_max
  Gain1 : Gain  Gain=1/(tg_max*tg_max)
  Math Function : Math
  Product : Product  Inputs=4
  p(t) : Outport
  wires:
  Constant/1 -> Product/1
  Constant1/1 -> Product/2
  Clock/1 -> Gain/1, Product/3
  Gain/1 -> Math Function/1
  Math Function/1 -> Product/4
  Product/1 -> Gain1/1
  Gain1/1 -> p(t)/1

== system estimator_de_stare/perturbatie12 ==
  Clock : Clock
  Constant : Constant  Value=Dg
  Constant1 : Constant  Value=Ag
  Gain : Gain  Gain=-1/tg_max
  Gain1 : Gain  Gain=1/(tg_max*tg_max)
  Math Function : Math
  Product : Product  Inputs=4
  p(t) : Outport
  wires:
  Constant/1 -> Product/1
  Constant1/1 -> Product/2
  Clock/1 -> Gain/1, Product/3
  Gain/1 -> Math Function/1
  Math Function/1 -> Product/4
  Product/1 -> Gain1/1
  Gain1/1 -> p(t)/1

== system estimator_de_stare/perturbatie13 ==
  Clock : Clock
  Constant : Constant  Value=Dg
  Constant1 : Constant  Value=Ag
  Gain : Gain  Gain=-1/tg_max
  Gain1 : Gain  Gain=1/(tg_max*tg_max)
  Math Function : Math
  Product : Product  Inputs=4
  p(t) : Outport
  wires:
  Constant/1 -> Product/1
  Constant1/1 -> Product/2
  Clock/1 -> Gain/1, Product/3
  Gain/1 -> Math Function/1
  Math Function/1 -> Product/4
  Product/1 -> Gain1/1
  Gain1/1 -> p(t)/1

== system estimator_de_stare/perturbatie8 ==
  Clock : Clock
  Constant : Constant  Value=Dg
  Constant1 : Constant  Value=Ag
  Gain : Gain  Gain=-1/tg_max
  Gain1 : Gain  Gain=1/(tg_max*tg_max)
  Math Function : Math
  Product : Product  Inputs=4
  p(t) : Outport
  wires:
  Constant/1 -> Product/1
  Constant1/1 -> Product/2
  Clock/1 -> Gain/1, Product/3
  Gain/1 -> Math Function/1
  Math Function/1 -> Product/4
  Product/1 -> Gain1/1
  Gain1/1 -> p(t)/1
